simulink model "Proyecto"  (R2023a)
settings: Solver=VariableStepAuto  StartTime=0.0  StopTime=1000000  RelTol=1e-3
settings Model: Creator=laura  LastModifiedBy=laura

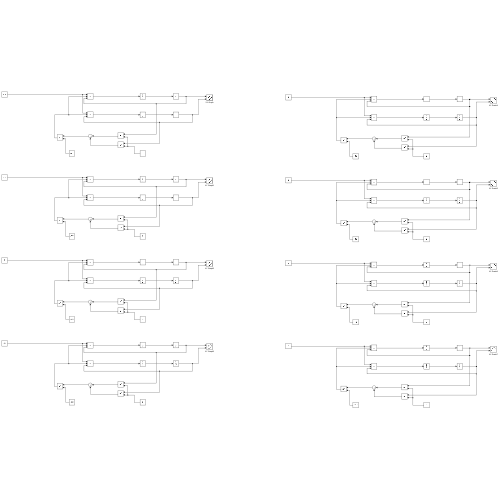
[thumbnail: Simulink's stored preview of the top-level diagram]
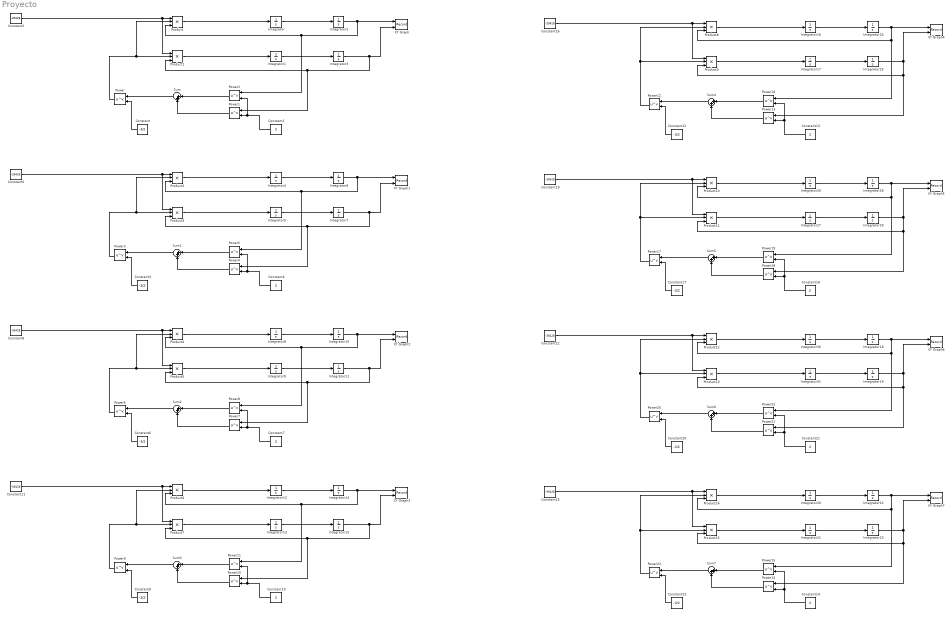
== system Proyecto ==
  Constant{,3,6,9,12,17,20,23} (8 alike) : Constant  Value=-3/2
  Constant{1,4,7,10,13..14,18,21} (8 alike) : Constant  Value=2
  Constant{2,5,8,11,15..16,19,22} (8 alike) : Constant  Value=-39428
  Integrator{,1,4..5,8..9,12..13,16..17,20..21,26..27,30..31} (16 alike) : Integrator  InitialCondition=-1
  Integrator{2,6,10,14,18,22,24,28} (8 alike) : Integrator
  Integrator11 : Integrator  InitialCondition=10000
  Integrator15 : Integrator  InitialCondition=15236
  Integrator19 : Integrator  InitialCondition=19192
  Integrator23 : Integrator  InitialCondition=30068
  Integrator25 : Integrator  InitialCondition=5200
  Integrator29 : Integrator  InitialCondition=9542
  Integrator3 : Integrator  InitialCondition=38700
  Integrator7 : Integrator  InitialCondition=7233
  Power{,1..23} (24 alike) : Math  Operator=pow
  Product{,1..15} (16 alike) : Product  Inputs=3
  Sum{,1..7} (8 alike) : Sum  Inputs=|++
  XY Graph : Record  FileSettingsInternal="{\"entries\":[{\"content\":{\"excelSettings\":{\"content\":{},\"type\":\"Streamout.ExcelSettings\"}},\"type\":\"Streamout.FileSettingStorage\",\"uuid\":\"df1110fe-10e8-4fe4-90f3-fcd62009f48e\"}],\"packageUris\":[\"http://schema.mathworks.com/mf0/streamout_blocks/R2020a\"],\"version\":\"1.0\"}"  Layout=[1 1]  SignalsInternal="{\"entries\":[{\"content\":{\"signals\":[{\"content\":{\"blockPath\":[\"Proyecto/XY Graph\"],\"dimensions\":[1],\"domain\":\"Proyecto/XY Graph\",\"lineColor\":\"#a2142f\",\"plots\":[1],\"port\":1,\"sid\":[\"\"],\"signalID\":2457,\"signalName\":\"Integrator2\"},\"type\":\"RecordBlkView.Signal\",\"uuid\":\"7a612d3a-345c-4701-8eab-9b103e7b2af3\"},{\"content\":{\"blockPath\":[\"Proyecto/XY Graph\"],\"dimensions\":[1],\"domain\":\"Proyecto/XY Graph\",\"lineColor\":\"#139fff\",\"plots\":[1],\"port\":2,\"sid\":[\"\"],\"signalID\":2461,\"signalName\":\"Integrator3\"},\"type\":\"RecordBlkView.Signal\",\"uuid\":\"e6806473-123f-4c44-a5f1-4c7375931891\"}]},\"type\":\"RecordBlkView.InputSignals\",\"uuid\":\"fe2a16fa-19bf-499f-ac8b-e8b5edca257b\"}],\"packageUris\":[\"http://schema.mathworks.com/mf0/streamout_blocks/R2020a\"],\"version\":\"1.0\"}"  VisualizationBindings="{\"xyplotplugin\":{\"info\":[{\"series\":[{\"bindingParametersList\":[{\"parameter\":\"X-Axis\",\"signalID\":2457,\"signalName\":\"Integrator2\"},{\"parameter\":\"Y-Axis\",\"signalID\":2461,\"signalName\":\"Integrator3\"}],\"seriesID\":21134}],\"subplotID\":1}]}}"  CompatibilityTag=XY
  XY Graph1 : Record  FileSettingsInternal="{\"entries\":[{\"content\":{\"excelSettings\":{\"content\":{},\"type\":\"Streamout.ExcelSettings\"}},\"type\":\"Streamout.FileSettingStorage\",\"uuid\":\"c4dfe1a7-50c7-47ec-b1e7-8a4068ecacfa\"}],\"packageUris\":[\"http://schema.mathworks.com/mf0/streamout_blocks/R2020a\"],\"version\":\"1.0\"}"  Layout=[1 1]  SignalsInternal="{\"entries\":[{\"content\":{\"signals\":[{\"content\":{\"blockPath\":[\"Proyecto/XY Graph1\"],\"dimensions\":[1],\"domain\":\"Proyecto/XY Graph1\",\"lineColor\":\"#a2142f\",\"plots\":[1],\"port\":1,\"sid\":[\"\"],\"signalID\":2505,\"signalName\":\"Integrator6\"},\"type\":\"RecordBlkView.Signal\",\"uuid\":\"49f4c184-6ebf-4cb2-a5ca-2a96d54003b5\"},{\"content\":{\"blockPath\":[\"Proyecto/XY Graph1\"],\"dimensions\":[1],\"domain\":\"Proyecto/XY Graph1\",\"lineColor\":\"#139fff\",\"plots\":[1],\"port\":2,\"sid\":[\"\"],\"signalID\":2509,\"signalName\":\"Integrator7\"},\"type\":\"RecordBlkView.Signal\",\"uuid\":\"8f9575a8-550a-466d-bba9-6736f03c81d1\"}]},\"type\":\"RecordBlkView.InputSignals\",\"uuid\":\"51204a3b-37a7-414c-8a33-25b85dcc383c\"}],\"packageUris\":[\"http://schema.mathworks.com/mf0/streamout_blocks/R2020a\"],\"version\":\"1.0\"}"  VisualizationBindings="{\"xyplotplugin\":{\"info\":[{\"series\":[{\"bindingParametersList\":[{\"parameter\":\"X-Axis\",\"signalID\":2505,\"signalName\":\"Integrator6\"},{\"parameter\":\"Y-Axis\",\"signalID\":2509,\"signalName\":\"Integrator7\"}],\"seriesID\":18238}],\"subplotID\":1}]}}"  CompatibilityTag=XY
  XY Graph2 : Record  FileSettingsInternal="{\"entries\":[{\"content\":{\"excelSettings\":{\"content\":{},\"type\":\"Streamout.ExcelSettings\"}},\"type\":\"Streamout.FileSettingStorage\",\"uuid\":\"4dd1dc28-af3b-4434-9179-1a2ddc6999fa\"}],\"packageUris\":[\"http://schema.mathworks.com/mf0/streamout_blocks/R2020a\"],\"version\":\"1.0\"}"  Layout=[1 1]  SignalsInternal="{\"entries\":[{\"content\":{\"signals\":[{\"content\":{\"blockPath\":[\"Proyecto/XY Graph2\"],\"dimensions\":[1],\"domain\":\"Proyecto/XY Graph2\",\"lineColor\":\"#a2142f\",\"plots\":[1],\"port\":1,\"sid\":[\"\"],\"signalID\":2513,\"signalName\":\"Integrator10\"},\"type\":\"RecordBlkView.Signal\",\"uuid\":\"d4489a48-e3c4-4438-9802-68ab23063581\"},{\"content\":{\"blockPath\":[\"Proyecto/XY Graph2\"],\"dimensions\":[1],\"domain\":\"Proyecto/XY Graph2\",\"lineColor\":\"#139fff\",\"plots\":[1],\"port\":2,\"sid\":[\"\"],\"signalID\":2517,\"signalName\":\"Integrator11\"},\"type\":\"RecordBlkView.Signal\",\"uuid\":\"10240eca-a5c9-4008-b7fd-849417d94ef5\"}]},\"type\":\"RecordBlkView.InputSignals\",\"uuid\":\"9de196f1-57e6-46c6-b1ea-81c30f3e2372\"}],\"packageUris\":[\"http://schema.mathworks.com/mf0/streamout_blocks/R2020a\"],\"version\":\"1.0\"}"  VisualizationBindings="{\"xyplotplugin\":{\"info\":[{\"series\":[{\"bindingParametersList\":[{\"parameter\":\"X-Axis\",\"signalID\":2513,\"signalName\":\"Integrator10\"},{\"parameter\":\"Y-Axis\",\"signalID\":2517,\"signalName\":\"Integrator11\"}],\"seriesID\":49025}],\"subplotID\":1}]}}"  CompatibilityTag=XY
  XY Graph3 : Record  FileSettingsInternal="{\"entries\":[{\"content\":{\"excelSettings\":{\"content\":{},\"type\":\"Streamout.ExcelSettings\"}},\"type\":\"Streamout.FileSettingStorage\",\"uuid\":\"44963c94-ea38-45ed-a5e6-49478b17dbd1\"}],\"packageUris\":[\"http://schema.mathworks.com/mf0/streamout_blocks/R2020a\"],\"version\":\"1.0\"}"  Layout=[1 1]  SignalsInternal="{\"entries\":[{\"content\":{\"signals\":[{\"content\":{\"blockPath\":[\"Proyecto/XY Graph3\"],\"dimensions\":[1],\"domain\":\"Proyecto/XY Graph3\",\"lineColor\":\"#a2142f\",\"plots\":[1],\"port\":1,\"sid\":[\"\"],\"signalID\":2465,\"signalName\":\"Integrator14\"},\"type\":\"RecordBlkView.Signal\",\"uuid\":\"f4ba95cb-00c2-40d7-ad34-24921cc250d5\"},{\"content\":{\"blockPath\":[\"Proyecto/XY Graph3\"],\"dimensions\":[1],\"domain\":\"Proyecto/XY Graph3\",\"lineColor\":\"#139fff\",\"plots\":[1],\"port\":2,\"sid\":[\"\"],\"signalID\":2469,\"signalName\":\"Integrator15\"},\"type\":\"RecordBlkView.Signal\",\"uuid\":\"b79d7d2a-4292-43c4-b365-57badb731545\"}]},\"type\":\"RecordBlkView.InputSignals\",\"uuid\":\"02a555a5-3c90-4653-8080-1bb8ed6bf6ac\"}],\"packageUris\":[\"http://schema.mathworks.com/mf0/streamout_blocks/R2020a\"],\"version\":\"1.0\"}"  VisualizationBindings="{\"xyplotplugin\":{\"info\":[{\"series\":[{\"bindingParametersList\":[{\"parameter\":\"X-Axis\",\"signalID\":2465,\"signalName\":\"Integrator14\"},{\"parameter\":\"Y-Axis\",\"signalID\":2469,\"signalName\":\"Integrator15\"}],\"seriesID\":10745}],\"subplotID\":1}]}}"  CompatibilityTag=XY
  XY Graph4 : Record  FileSettingsInternal="{\"entries\":[{\"content\":{\"excelSettings\":{\"content\":{},\"type\":\"Streamout.ExcelSettings\"}},\"type\":\"Streamout.FileSettingStorage\",\"uuid\":\"e36909f4-f642-4b54-899f-5f2f6e84cfd9\"}],\"packageUris\":[\"http://schema.mathworks.com/mf0/streamout_blocks/R2020a\"],\"version\":\"1.0\"}"  Layout=[1 1]  SignalsInternal="{\"entries\":[{\"content\":{\"signals\":[{\"content\":{\"blockPath\":[\"Proyecto/XY Graph4\"],\"dimensions\":[1],\"domain\":\"Proyecto/XY Graph4\",\"lineColor\":\"#a2142f\",\"plots\":[1],\"port\":1,\"sid\":[\"\"],\"signalID\":2473,\"signalName\":\"Integrator24\"},\"type\":\"RecordBlkView.Signal\",\"uuid\":\"54657030-c10e-4710-9f1f-640cdc790c5a\"},{\"content\":{\"blockPath\":[\"Proyecto/XY Graph4\"],\"dimensions\":[1],\"domain\":\"Proyecto/XY Graph4\",\"lineColor\":\"#139fff\",\"plots\":[1],\"port\":2,\"sid\":[\"\"],\"signalID\":2477,\"signalName\":\"Integrator25\"},\"type\":\"RecordBlkView.Signal\",\"uuid\":\"92f0ec25-6d80-462d-8d4b-764dbe2d5e4c\"}]},\"type\":\"RecordBlkView.InputSignals\",\"uuid\":\"aa6dda34-5227-4e26-9685-ab603c988471\"}],\"packageUris\":[\"http://schema.mathworks.com/mf0/streamout_blocks/R2020a\"],\"version\":\"1.0\"}"  VisualizationBindings="{\"xyplotplugin\":{\"info\":[{\"series\":[{\"bindingParametersList\":[{\"parameter\":\"X-Axis\",\"signalID\":2473,\"signalName\":\"Integrator24\"},{\"parameter\":\"Y-Axis\",\"signalID\":2477,\"signalName\":\"Integrator25\"}],\"seriesID\":20310}],\"subplotID\":1}]}}"  CompatibilityTag=XY
  XY Graph5 : Record  FileSettingsInternal="{\"entries\":[{\"content\":{\"excelSettings\":{\"content\":{},\"type\":\"Streamout.ExcelSettings\"}},\"type\":\"Streamout.FileSettingStorage\",\"uuid\":\"06fc2b16-290e-4a7d-af9f-2a490dba25d6\"}],\"packageUris\":[\"http://schema.mathworks.com/mf0/streamout_blocks/R2020a\"],\"version\":\"1.0\"}"  Layout=[1 1]  SignalsInternal="{\"entries\":[{\"content\":{\"signals\":[{\"content\":{\"blockPath\":[\"Proyecto/XY Graph5\"],\"dimensions\":[1],\"domain\":\"Proyecto/XY Graph5\",\"lineColor\":\"#a2142f\",\"plots\":[1],\"port\":1,\"sid\":[\"\"],\"signalID\":2489,\"signalName\":\"Integrator28\"},\"type\":\"RecordBlkView.Signal\",\"uuid\":\"902b754d-5e6f-49c6-b638-ca19866bff63\"},{\"content\":{\"blockPath\":[\"Proyecto/XY Graph5\"],\"dimensions\":[1],\"domain\":\"Proyecto/XY Graph5\",\"lineColor\":\"#139fff\",\"plots\":[1],\"port\":2,\"sid\":[\"\"],\"signalID\":2493,\"signalName\":\"Integrator29\"},\"type\":\"RecordBlkView.Signal\",\"uuid\":\"52cdd28a-99e3-4cf9-8d1e-b9c14f6f4d60\"}]},\"type\":\"RecordBlkView.InputSignals\",\"uuid\":\"223f4df8-7fd4-4861-b98f-c792a4c63ca3\"}],\"packageUris\":[\"http://schema.mathworks.com/mf0/streamout_blocks/R2020a\"],\"version\":\"1.0\"}"  VisualizationBindings="{\"xyplotplugin\":{\"info\":[{\"series\":[{\"bindingParametersList\":[{\"parameter\":\"X-Axis\",\"signalID\":2489,\"signalName\":\"Integrator28\"},{\"parameter\":\"Y-Axis\",\"signalID\":2493,\"signalName\":\"Integrator29\"}],\"seriesID\":21301}],\"subplotID\":1}]}}"  CompatibilityTag=XY
  XY Graph6 : Record  FileSettingsInternal="{\"entries\":[{\"content\":{\"excelSettings\":{\"content\":{},\"type\":\"Streamout.ExcelSettings\"}},\"type\":\"Streamout.FileSettingStorage\",\"uuid\":\"c78ec36a-7255-4aae-ae4f-8be4809e378d\"}],\"packageUris\":[\"http://schema.mathworks.com/mf0/streamout_blocks/R2020a\"],\"version\":\"1.0\"}"  Layout=[1 1]  SignalsInternal="{\"entries\":[{\"content\":{\"signals\":[{\"content\":{\"blockPath\":[\"Proyecto/XY Graph6\"],\"dimensions\":[1],\"domain\":\"Proyecto/XY Graph6\",\"lineColor\":\"#a2142f\",\"plots\":[1],\"port\":1,\"sid\":[\"\"],\"signalID\":2497,\"signalName\":\"Integrator18\"},\"type\":\"RecordBlkView.Signal\",\"uuid\":\"a0f47ddc-25cb-4db9-8dba-e48e47a79aa6\"},{\"content\":{\"blockPath\":[\"Proyecto/XY Graph6\"],\"dimensions\":[1],\"domain\":\"Proyecto/XY Graph6\",\"lineColor\":\"#139fff\",\"plots\":[1],\"port\":2,\"sid\":[\"\"],\"signalID\":2501,\"signalName\":\"Integrator19\"},\"type\":\"RecordBlkView.Signal\",\"uuid\":\"dee557ae-58ab-4868-bfa6-9a89b8f9b5a7\"}]},\"type\":\"RecordBlkView.InputSignals\",\"uuid\":\"b043698c-5f14-4085-98bf-77b09a583f83\"}],\"packageUris\":[\"http://schema.mathworks.com/mf0/streamout_blocks/R2020a\"],\"version\":\"1.0\"}"  VisualizationBindings="{\"xyplotplugin\":{\"info\":[{\"series\":[{\"bindingParametersList\":[{\"parameter\":\"X-Axis\",\"signalID\":2497,\"signalName\":\"Integrator18\"},{\"parameter\":\"Y-Axis\",\"signalID\":2501,\"signalName\":\"Integrator19\"}],\"seriesID\":39091}],\"subplotID\":1}]}}"  CompatibilityTag=XY
  XY Graph7 : Record  FileSettingsInternal="{\"entries\":[{\"content\":{\"excelSettings\":{\"content\":{},\"type\":\"Streamout.ExcelSettings\"}},\"type\":\"Streamout.FileSettingStorage\",\"uuid\":\"989537d0-db8b-470e-b695-49cf62161d3b\"}],\"packageUris\":[\"http://schema.mathworks.com/mf0/streamout_blocks/R2020a\"],\"version\":\"1.0\"}"  Layout=[1 1]  SignalsInternal="{\"entries\":[{\"content\":{\"signals\":[{\"content\":{\"blockPath\":[\"Proyecto/XY Graph7\"],\"dimensions\":[1],\"domain\":\"Proyecto/XY Graph7\",\"lineColor\":\"#a2142f\",\"plots\":[1],\"port\":1,\"sid\":[\"\"],\"signalID\":2481,\"signalName\":\"Integrator22\"},\"type\":\"RecordBlkView.Signal\",\"uuid\":\"8d823806-4507-43dd-8df7-1530f14791f9\"},{\"content\":{\"blockPath\":[\"Proyecto/XY Graph7\"],\"dimensions\":[1],\"domain\":\"Proyecto/XY Graph7\",\"lineColor\":\"#139fff\",\"plots\":[1],\"port\":2,\"sid\":[\"\"],\"signalID\":2485,\"signalName\":\"Integrator23\"},\"type\":\"RecordBlkView.Signal\",\"uuid\":\"8540591e-3093-4697-8451-d031ecd479e8\"}]},\"type\":\"RecordBlkView.InputSignals\",\"uuid\":\"ef47d085-3e6d-48fb-bb10-5795ecdba0bd\"}],\"packageUris\":[\"http://schema.mathworks.com/mf0/streamout_blocks/R2020a\"],\"version\":\"1.0\"}"  VisualizationBindings="{\"xyplotplugin\":{\"info\":[{\"series\":[{\"bindingParametersList\":[{\"parameter\":\"X-Axis\",\"signalID\":2481,\"signalName\":\"Integrator22\"},{\"parameter\":\"Y-Axis\",\"signalID\":2485,\"signalName\":\"Integrator23\"}],\"seriesID\":5067}],\"subplotID\":1}]}}"  CompatibilityTag=XY
  wires:
  Sum/1 -> Power/1
  Power2/1 -> Sum/1
  Power1/1 -> Sum/2
  Constant1/1 -> Power2/2, Power1/2
  Constant/1 -> Power/2
  Power/1 -> Product1/2, Product/2
  Integrator/1 -> Integrator2/1
  Integrator1/1 -> Integrator3/1
  Integrator2/1 -> Power2/1, Product/3, XY Graph/1
  Integrator3/1 -> XY Graph/2, Power1/1, Product1/3
  Constant2/1 -> Product1/1, Product/1
  Product/1 -> Integrator/1
  Product1/1 -> Integrator1/1
  Constant3/1 -> Power3/2
  Integrator5/1 -> Integrator7/1
  Product2/1 -> Integrator4/1
  Sum1/1 -> Power3/1
  Product3/1 -> Integrator5/1
  Integrator4/1 -> Integrator6/1
  Constant4/1 -> Power5/2, Power4/2
  Integrator6/1 -> Power5/1, Product2/3, XY Graph1/1
  Power3/1 -> Product3/2, Product2/2
  Constant5/1 -> Product3/1, Product2/1
  Integrator7/1 -> XY Graph1/2, Power4/1, Product3/3
  Power5/1 -> Sum1/1
  Power4/1 -> Sum1/2
  Power8/1 -> Sum2/1
  Constant8/1 -> Product5/1, Product4/1
  Integrator10/1 -> Power8/1, Product4/3, XY Graph2/1
  Integrator11/1 -> XY Graph2/2, Power7/1, Product5/3
  Integrator9/1 -> Integrator11/1
  Constant6/1 -> Power6/2
  Integrator8/1 -> Integrator10/1
  Power7/1 -> Sum2/2
  Product4/1 -> Integrator8/1
  Sum2/1 -> Power6/1
  Constant7/1 -> Power8/2, Power7/2
  Power6/1 -> Product5/2, Product4/2
  Product5/1 -> Integrator9/1
  Power11/1 -> Sum3/1
  Constant11/1 -> Product7/1, Product6/1
  Integrator14/1 -> Power11/1, Product6/3, XY Graph3/1
  Integrator15/1 -> XY Graph3/2, Power10/1, Product7/3
  Integrator13/1 -> Integrator15/1
  Constant9/1 -> Power9/2
  Integrator12/1 -> Integrator14/1
  Power10/1 -> Sum3/2
  Product6/1 -> Integrator12/1
  Sum3/1 -> Power9/1
  Constant10/1 -> Power11/2, Power10/2
  Power9/1 -> Product7/2, Product6/2
  Product7/1 -> Integrator13/1
  Integrator30/1 -> Integrator18/1
  Power21/1 -> Sum6/2
  Product10/1 -> Integrator26/1
  Constant22/1 -> Product13/1, Product12/1
  Constant20/1 -> Power20/2
  Integrator26/1 -> Integrator28/1
  Constant17/1 -> Power17/2
  Constant23/1 -> Power23/2
  Constant19/1 -> Product11/1, Product10/1
  Sum5/1 -> Power17/1
  Integrator27/1 -> Integrator29/1
  Product13/1 -> Integrator31/1
  Integrator19/1 -> XY Graph6/2, Power21/1, Product13/3
  Power13/1 -> Sum4/2
  Power20/1 -> Product13/2, Product12/2
  Constant16/1 -> Product9/1, Product8/1
  Power14/1 -> Sum7/2
  Constant13/1 -> Power16/2, Power13/2
  Integrator24/1 -> Power16/1, Product8/3, XY Graph4/1
  Integrator18/1 -> Power22/1, Product12/3, XY Graph6/1
  Integrator16/1 -> Integrator24/1
  Power19/1 -> Sum5/1
  Power22/1 -> Sum6/1
  Sum4/1 -> Power12/1
  Power16/1 -> Sum4/1
  Integrator31/1 -> Integrator19/1
  Power15/1 -> Sum7/1
  Product8/1 -> Integrator16/1
  Product9/1 -> Integrator17/1
  Product12/1 -> Integrator30/1
  Integrator22/1 -> Power15/1, Product14/3, XY Graph7/1
  Integrator28/1 -> Power19/1, Product10/3, XY Graph5/1
  Product14/1 -> Integrator20/1
  Integrator20/1 -> Integrator22/1
  Integrator29/1 -> XY Graph5/2, Power18/1, Product11/3
  Power12/1 -> Product9/2, Product8/2
  Sum6/1 -> Power20/1
  Power17/1 -> Product11/2, Product10/2
  Product11/1 -> Integrator27/1
  Sum7/1 -> Power23/1
  Constant15/1 -> Product15/1, Product14/1
  Product15/1 -> Integrator21/1
  Integrator21/1 -> Integrator23/1
  Constant18/1 -> Power19/2, Power18/2
  Power18/1 -> Sum5/2
  Constant21/1 -> Power22/2, Power21/2
  Integrator17/1 -> Integrator25/1
  Constant12/1 -> Power12/2
  Power23/1 -> Product15/2, Product14/2
  Integrator23/1 -> XY Graph7/2, Power14/1, Product15/3
  Constant14/1 -> Power15/2, Power14/2
  Integrator25/1 -> XY Graph4/2, Power13/1, Product9/3
